simulink model "EINT_system_simulation"  (R2025b)
settings: Solver=FixedStepAuto  StartTime=0.0  StopTime=15  FixedStep=Ts  RelTol=1e-3
values from neighbouring files (symbols this model uses):
  nx = nx_nn + nx_phy    (= 18)    [MPC_NN.m]
  Ts = 0.05    [MPC_NN.m]    (also in UAV_StateTransitionFcn.m; random_init.m)
libraries: sharedTrackingLibrary x1, mpclib x1
settings Model: Creator=Max  LastModifiedBy=baolgr
settings SolverCC: AlgebraicLoopSolver=TrustRegion
settings DebuggingCC: UnconnectedInputMsg=warning  UnconnectedOutputMsg=warning  UnconnectedLineMsg=warning
settings ModelReferenceCC: EnableRefExpFcnMdlSchedulingChecks=on
settings RTWCC: GPUComputeCapability=3.5

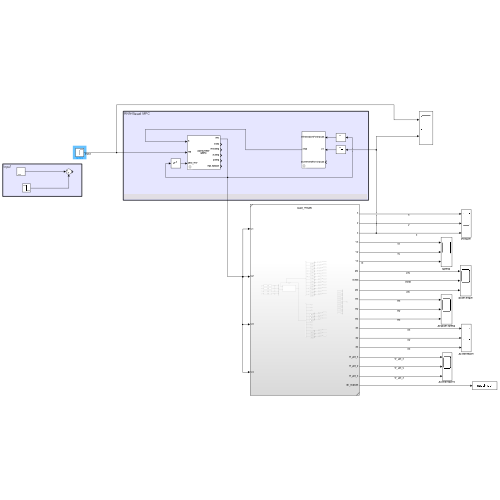
[thumbnail: Simulink's stored preview of the top-level diagram]
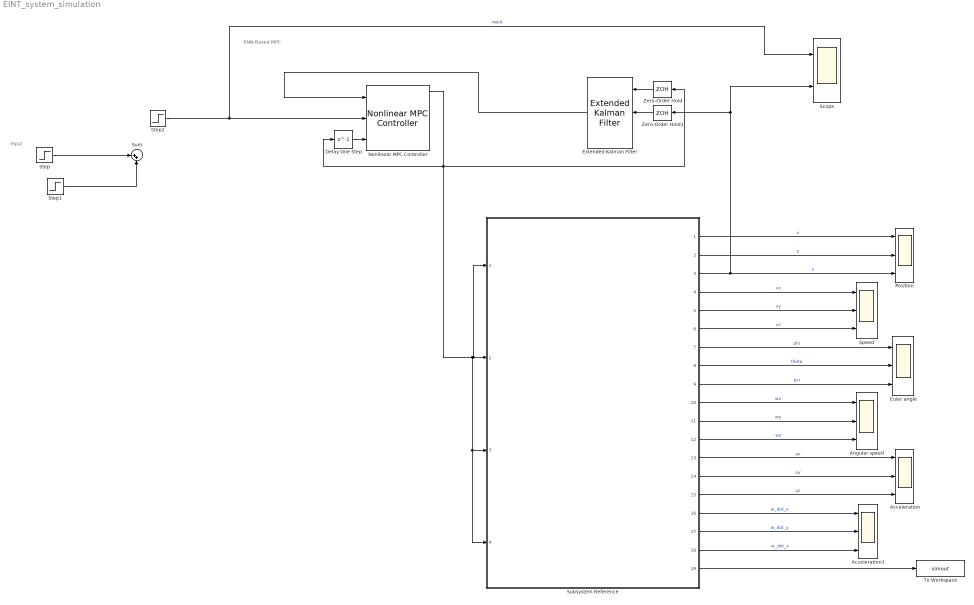
== system EINT_system_simulation ==
  note: RNN-Based MPC
  note: Input
  Acceleration : Scope  NumInputPorts=3
      settings: ActiveDisplayYMinimum=-35.48317  ActiveDisplayYMaximum=15.8515
  Acceleration1 : Scope  NumInputPorts=3
      settings: ActiveDisplayYMinimum=-1052.98102  ActiveDisplayYMaximum=116.99789  DataLoggingVariableName=ScopeData2
  Angular speed : Scope  NumInputPorts=3
      settings: ActiveDisplayYMinimum=-0.45167  ActiveDisplayYMaximum=0.49611  DataLoggingVariableName=ScopeData3
  Delay One Step : Delay  DelayLength=1
  Euler angle : Scope  NumInputPorts=3
      settings: ActiveDisplayYMinimum=-1695.66598  ActiveDisplayYMaximum=1344.64163  DataLoggingVariableName=ScopeData4
  Extended Kalman Filter : sharedTrackingLibrary/Extended Kalman Filter  StateTransitionFcn=UAV_StateTransitionFcn  HasStateTransitionJacobianFcn=off  HasAdditiveProcessNoise=Additive  ProcessNoise=0.1  HasTimeVaryingProcessNoise=off  HasStateTransitionFcnExtraArgument=1  InitialState=zeros(nx,1)  InitialStateCovariance=1  MeasurementFcn1=UAV_MeasurementFcn  HasMeasurementJacobianFcn1=off  HasMeasurementEnablePort1=off  HasAdditiveMeasurementNoise1=Additive  MeasurementNoise1=0.1  HasTimeVaryingMeasurementNoise1=off  HasMeasurementFcnExtraArgument1=1  HasMeasurementWrapping1=off  MeasurementFcn2=myMeasurementFcn  HasMeasurementJacobianFcn2=off  HasMeasurementEnablePort2=off  HasAdditiveMeasurementNoise2=Additive  MeasurementNoise2=1  HasTimeVaryingMeasurementNoise2=off  HasMeasurementFcnExtraArgument2=0  HasMeasurementWrapping2=off  MeasurementFcn3=myMeasurementFcn  HasMeasurementJacobianFcn3=off  HasMeasurementEnablePort3=off  HasAdditiveMeasurementNoise3=Additive  MeasurementNoise3=1  HasTimeVaryingMeasurementNoise3=off  HasMeasurementFcnExtraArgument3=0  HasMeasurementWrapping3=off  MeasurementFcn4=myMeasurementFcn  HasMeasurementJacobianFcn4=off  HasMeasurementEnablePort4=off  HasAdditiveMeasurementNoise4=Additive  MeasurementNoise4=1  HasTimeVaryingMeasurementNoise4=off  HasMeasurementFcnExtraArgument4=0  HasMeasurementWrapping4=off  MeasurementFcn5=myMeasurementFcn  HasMeasurementJacobianFcn5=off  HasMeasurementEnablePort5=off  HasAdditiveMeasurementNoise5=Additive  MeasurementNoise5=1  HasTimeVaryingMeasurementNoise5=off  HasMeasurementFcnExtraArgument5=0  HasMeasurementWrapping5=off  EnableMultirate=off  StateTransitionFcnSampleTime=1  MeasurementFcn1SampleTime=1  MeasurementFcn2SampleTime=1  MeasurementFcn3SampleTime=1  MeasurementFcn4SampleTime=1  MeasurementFcn5SampleTime=1  UseCurrentEstimator=on  OutputStateCovariance=off  DataType=double  SampleTime=Ts  NumberOfMeasurements=1
  Nonlinear MPC Controller : mpclib/Nonlinear MPC Controller  nlmpcobj=nlmpc_nn  UseObjectTs=on  UseMEX=off  md_enabled=off  mvtarget_enabled=off  param_enabled=off  cost_enabled=on  mvseq_enabled=on  stateseq_enabled=on  ovseq_enabled=on  slack_enabled=off  status_enabled=on  ov_min=off  ov_max=off  mv_min=off  mv_max=off  mvrate_min=off  mvrate_max=off  state_min=off  state_max=off  ov_weight=off  mv_weight=off  mvrate_weight=off  ecr_weight=off  nlp_initialize=off
  Position : Scope  NumInputPorts=3
      settings: ActiveDisplayYMinimum=-186.84870127715556  ActiveDisplayYMaximum=80.469634317250083  DataLoggingVariableName=ScopeData6
  Scope : Scope  NumInputPorts=2
      settings: ActiveDisplayYMinimum=-102.5438005692626  ActiveDisplayYMaximum=136.58776419367197  DataLoggingVariableName=ScopeData5
  Speed : Scope  NumInputPorts=3
      settings: ActiveDisplayYMinimum=-1193.81123  ActiveDisplayYMaximum=133.09449
  Step : Step  After=50  SampleTime=0
  Step1 : Step  Time=15  After=-75  SampleTime=0
  Step2 : Step  After=100  SampleTime=0
  Subsystem Reference : Subsystem  ReferencedSubsystem=UAV_model
  Sum : Sum  Inputs=|++
  To Workspace : ToWorkspace  VariableName=simout  SaveFormat=Structure With Time  SampleTime=Ts
  Zero-Order Hold : ZeroOrderHold  SampleTime=Ts
  Zero-Order Hold1 : ZeroOrderHold  SampleTime=Ts
  wires:
  Subsystem Reference/18 -> Acceleration1/3  "w_dot_z"
  Subsystem Reference/12 -> Angular speed/3  "wz"
  Subsystem Reference/17 -> Acceleration1/2  "w_dot_y"
  Subsystem Reference/9 -> Euler angle/3  "psi"
  Subsystem Reference/8 -> Euler angle/2  "theta"
  Subsystem Reference/14 -> Acceleration/2  "ay"
  Subsystem Reference/10 -> Angular speed/1  "wx"
  Subsystem Reference/2 -> Position/2  "y"
  Subsystem Reference/13 -> Acceleration/1  "ax"
  Subsystem Reference/15 -> Acceleration/3  "az"
  Subsystem Reference/16 -> Acceleration1/1  "w_dot_x"
  Subsystem Reference/7 -> Euler angle/1  "phi"
  Subsystem Reference/19 -> To Workspace/1
  Subsystem Reference/1 -> Position/1  "x"
  Subsystem Reference/6 -> Speed/3  "vz"
  Subsystem Reference/4 -> Speed/1  "vx"
  Subsystem Reference/3 -> Scope/2, Zero-Order Hold1/1, Position/3  "z"
  Subsystem Reference/5 -> Speed/2  "vy"
  Subsystem Reference/11 -> Angular speed/2  "wy"
  Nonlinear MPC Controller/1 -> Subsystem Reference/4, Subsystem Reference/3, Subsystem Reference/1, Subsystem Reference/2, Zero-Order Hold/1, Delay One Step/1
  Delay One Step/1 -> Nonlinear MPC Controller/3
  Extended Kalman Filter/1 -> Nonlinear MPC Controller/1
  Zero-Order Hold/1 -> Extended Kalman Filter/1
  Zero-Order Hold1/1 -> Extended Kalman Filter/2
  Step2/1 -> Scope/1, Nonlinear MPC Controller/2  "input"
  Step1/1 -> Sum/2
  Step/1 -> Sum/1
